simulink model "mpc_tgt_calc"  (R2025a)
settings: Solver=FixedStepDiscrete  StartTime=0.0  StopTime=2600  FixedStep=0.1  RelTol=1e-3
undefined symbols (not defined in the file): accl, alpha, alpha2, ang, beta, cnt_delay_accl_ratio, cnt_delay_decel_ratio, delay_accl, delay_v, dist, dt, ff_duty_front, ff_duty_l, ff_duty_r, ff_duty_roll, ff_duty_rpm_l, ff_duty_rpm_r, ff_friction_torque_l, ff_friction_torque_r, ff_front_torque, ff_roll_torque, ideal_point, img_ang, img_dist, kanayama_point, pivot_state, pos_x, pos_y, sla_param, slip, slip_point, state, trj_diff, v, vx, vy, w
libraries: simulink_extras x1
(part 1 of 3)
settings Model: Creator=nao12  LastModifiedBy=naoto
settings SolverCC: AlgebraicLoopSolver=TrustRegion
settings DataIOCC: SaveOutput=off  SignalLogging=off  DSMLogging=off  SaveTime=off  ReturnWorkspaceOutputs=off
settings OptimizationCC: StrengthReduction=on  PassReuseOutputArgsAs=Individual arguments  ZeroExternalMemoryAtStartup=off  ZeroInternalMemoryAtStartup=off  OptimizeBlockOrder=speed  OptimizationPriority=Speed  OptimizationCustomize=off  MultiThreadedLoops=on  AutoScheduleForLoops=on  EfficientTunableParamExpr=on
settings DebuggingCC: ParameterTunabilityLossMsg=error  UnconnectedInputMsg=warning  UnconnectedOutputMsg=warning  UnconnectedLineMsg=warning  ArithmeticOperatorsInVariantConditions=warning
settings ModelReferenceCC: EnableRefExpFcnMdlSchedulingChecks=on
settings SFSimCC: SimCustomHeaderCode="#include \"bus.h\""  SimUserIncludeDirs=../include/  MATLABDynamicMemAlloc=off  CustomCodeUndefinedFunction=UseInterfaceOnly  SimTargetLang=C++  SimDLTargetLibrary=mkl-dnn
settings RTWCC: SystemTargetFile=ert.tlc  GenCodeOnly=on  TemplateMakefile=ert_default_tmf  GenerateReport=on  RTWUseSimCustomCode=on  CustomHeaderCode="#include \"bus.h\""  CustomInclude=../include/  Toolchain=GNU gcc/g++ | gmake (64-bit Linux)  IncludeHyperlinkInReport=on  LaunchReport=on  TargetLang=C++  GenerateTraceInfo=on  GenerateTraceReport=on  GenerateTraceReportSl=on  GenerateTraceReportSf=on  GenerateTraceReportEml=on  GenerateCodeMetricsReport=on  GPUComputeCapability=3.5  DLArmComputeVersion=19.05  Description=Embedded Coder
settings CodeAppCC: GenerateComments=off  IgnoreCustomStorageClasses=off  OperatorAnnotations=on  SimulinkDataObjDesc=on  SFDataObjDesc=on  SimulinkBlockComments=off
settings ERTTargetCC: ExtModeTransport=0.0  ExtModeStaticAlloc=off  ExtModeMexFile=ext_comm  ExtModeIntrfLevel=Level1  InlinedParameterPlacement=Hierarchical  RootIOFormat=Structure reference  ERTCustomFileTemplate=example_file_process.tlc  DynamicArrayContainerType=coder::array  TargetLangStandard=C++11 (ISO)  GenerateSampleERTMain=on  SupportAbsoluteTime=off  CodeInterfacePackaging=C++ class  SupportComplex=off  ParenthesesLevel=Minimum
settings SimscapeCC: SimscapeLogDecimation=1  SimscapeLogDataHistory=5000

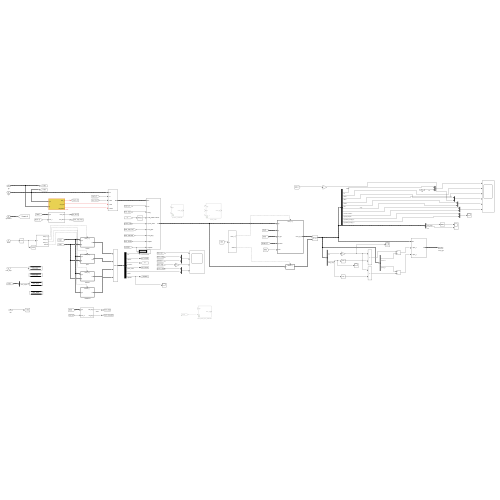
[thumbnail: Simulink's stored preview of the top-level diagram]
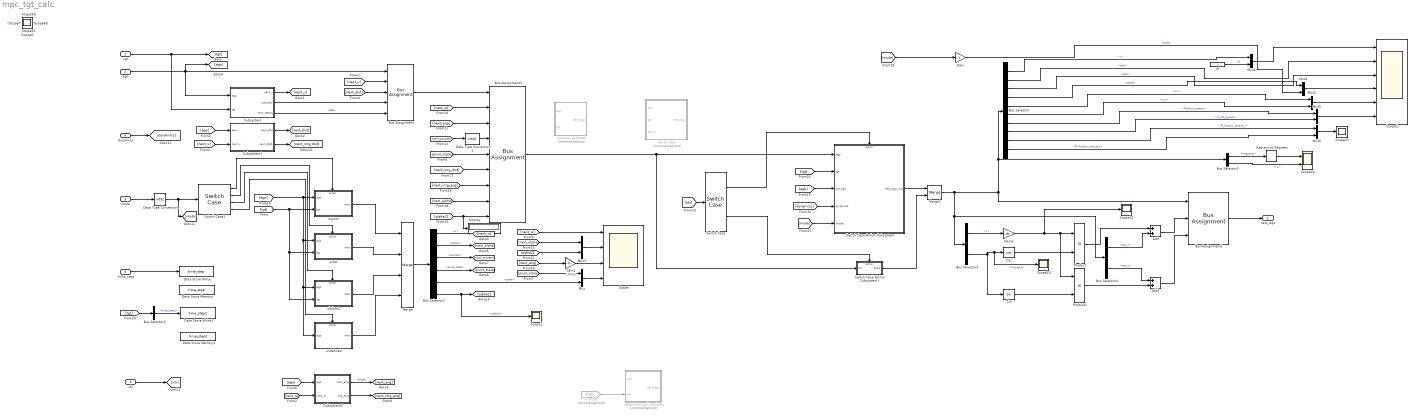
== system mpc_tgt_calc ==
  tgt : Inport  OutDataTypeStr=Bus: t_tgt  BusOutputAsStruct=on
  ego : Inport  Port=2  OutDataTypeStr=Bus: t_ego  BusOutputAsStruct=on
  mode : Inport  Port=3  OutDataTypeStr=int32
  time_step : Inport  Port=4  OutDataTypeStr=int32
  dynamics : Inport  Port=5  OutDataTypeStr=Bus: t_dynamics  BusOutputAsStruct=on
  idx : Inport  Port=6  OutDataTypeStr=int32
  Add : Sum
  Add1 : Sum
  Bus Assignment : BusAssignment  AssignedSignals=v,dist,accl,state
  Bus Assignment1 : BusAssignment  AssignedSignals=w,ang,sla_param.counter,pivot_state,img_dist,img_ang,alpha,alpha2
  Bus Assignment2 : BusAssignment  AssignedSignals=pos_x,pos_y
  Bus Selector : BusSelector  OutputSignals=v,accl,dist,state,slip.vx,slip.vy,ff_front_torque,ff_roll_torque,ff_friction_torque_l,ff_friction_torque_r
  Bus Selector1 : BusSelector  OutputSignals=w,alpha,sla_param.counter,pivot_state,sla_param.state,alpha2
  Bus Selector2 : BusSelector  OutputSignals=time_step2
  Bus Selector3 : BusSelector  OutputSignals=v,img_ang
  Bus Selector4 : BusSelector  OutputSignals=pos_x,pos_y
  Bus Selector5 : BusSelector  OutputSignals=img_ang,w
  Cos : Trigonometry  Operator=cos
  Data Store Memory : DataStoreMemory  DataStoreName=time_step  ReadBeforeWriteMsg=warning  WriteAfterWriteMsg=warning  WriteAfterReadMsg=warning  ShowAdditionalParam=off
  Data Store Memory1 : DataStoreMemory  DataStoreName=time_step2  ReadBeforeWriteMsg=warning  WriteAfterWriteMsg=warning  WriteAfterReadMsg=warning  ShowAdditionalParam=off
  Data Store Write : DataStoreWrite  DataStoreName=time_step  IndexOptions=Index vector (dialog)  Indices=1  OutputSizes=1
  Data Store Write1 : DataStoreWrite  DataStoreName=time_step2  IndexOptions=Index vector (dialog)  Indices=1  OutputSizes=1
  Data Type Conversion : DataTypeConversion  OutDataTypeStr=int32  SaturateOnIntegerOverflow=off  RndMeth=Floor
  Data Type Conversion1 : DataTypeConversion  OutDataTypeStr=int32  SaturateOnIntegerOverflow=off  RndMeth=Floor
  Display : Display
  From19 : From  Commented=on  GotoTag=tgt
  Gain : Gain  OutDataTypeStr=int32
  Gain1 : Gain  Gain=180/pi
  Gain2 : Gain  Gain=dt
  Merge : Merge  Inputs=4
  Merge1 : Merge
  Mux{,1..6} (7 alike) : Mux  Inputs=2
  Product : Product
  Product1 : Product
  Radians to Degrees : simulink_extras/Transformations/Radians to Degrees
  Scope : Scope  NumInputPorts=4
      settings: ActiveDisplayYMinimum=-2.63908  ActiveDisplayYMaximum=23.74994  DataLoggingVariableName=ScopeData2
  Scope{1,3..19,21..23} (21 alike) : Scope
      Scope1 settings: ActiveDisplayYMinimum=-2973.3984756469727  ActiveDisplayYMaximum=1247.0022964477539  DataLoggingVariableName=ScopeData2
      Scope21 settings: ActiveDisplayYMinimum=0.0163018349558115  ActiveDisplayYMaximum=0.017838163301348686
      Scope22 settings: ActiveDisplayYMinimum=0.20000004768371582  ActiveDisplayYMaximum=2.2000000476837158  DataLoggingVariableName=ScopeData10
      Scope23 settings: ActiveDisplayYMinimum=0.20000004768371582  ActiveDisplayYMaximum=2.2000000476837158  DataLoggingVariableName=ScopeData11
      Scope10 settings: ActiveDisplayYMinimum=0.5708  ActiveDisplayYMaximum=2.5708  DataLoggingVariableName=ScopeData3
      Scope11 settings: ActiveDisplayYMinimum=-360.06396  ActiveDisplayYMaximum=3240.57568  DataLoggingVariableName=ScopeData4
      Scope12 settings: ActiveDisplayYMinimum=1880  ActiveDisplayYMaximum=3880  DataLoggingVariableName=ScopeData5
      Scope13 settings: ActiveDisplayYMinimum=-0.97134  ActiveDisplayYMaximum=-0.37241  DataLoggingVariableName=ScopeData6
      Scope14 settings: ActiveDisplayYMinimum=-11.26948  ActiveDisplayYMaximum=1.25216  DataLoggingVariableName=ScopeData7
      Scope15 settings: DataLoggingVariableName=ScopeData8
      Scope16 settings: ActiveDisplayYMinimum=-1  ActiveDisplayYMaximum=1  DataLoggingVariableName=ScopeData9
      Scope17 settings: ActiveDisplayYMinimum=-22.53325  ActiveDisplayYMaximum=202.50369
      Scope18 settings: ActiveDisplayYMinimum=-1  ActiveDisplayYMaximum=1
      Scope19 settings: ActiveDisplayYMinimum=-0.125  ActiveDisplayYMaximum=1.125  DataLoggingVariableName=ScopeData2
      Scope3 settings: ActiveDisplayYMinimum=-11  ActiveDisplayYMaximum=-9  DataLoggingVariableName=ScopeData4
      Scope4 settings: ActiveDisplayYMinimum=-11  ActiveDisplayYMaximum=-9  DataLoggingVariableName=ScopeData5
      Scope5 settings: ActiveDisplayYMinimum=-11  ActiveDisplayYMaximum=-9  DataLoggingVariableName=ScopeData6
      Scope6 settings: ActiveDisplayYMinimum=9  ActiveDisplayYMaximum=11  DataLoggingVariableName=ScopeData7
      Scope7 settings: ActiveDisplayYMinimum=-1  ActiveDisplayYMaximum=1  DataLoggingVariableName=ScopeData8
      Scope8 settings: ActiveDisplayYMinimum=-0.25  ActiveDisplayYMaximum=2.25
      Scope9 settings: ActiveDisplayYMinimum=0.0004  ActiveDisplayYMaximum=0.0006  DataLoggingVariableName=ScopeData2
  Scope2 : Scope  NumInputPorts=6
      settings: ActiveDisplayYMinimum=-724.5  ActiveDisplayYMaximum=6520.5
  Scope20 : Scope  NumInputPorts=2
      settings: ActiveDisplayYMinimum=-5.62498  ActiveDisplayYMaximum=50.64557  DataLoggingVariableName=ScopeData2
  Sin : Trigonometry
  Subsystem : Subsystem
  Subsystem1 : Subsystem
  Subsystem3 : Subsystem
  Switch Case : SwitchCase
  Switch Case Action Subsystem : Subsystem  TreatAsAtomicUnit=on
  Switch Case Action Subsystem1 : Subsystem  TreatAsAtomicUnit=on
  Switch Case1 : SwitchCase  CaseConditions={1,2,4}
  decel_ratio : Subsystem  Commented=on
  kanayama_ctrl_method1 : Subsystem  Commented=on
  pivot : Subsystem  TreatAsAtomicUnit=on
  position_estimate : Subsystem  Commented=on
  slalom : Subsystem  TreatAsAtomicUnit=on
  slalom2 : Subsystem  TreatAsAtomicUnit=on
  undefined : Subsystem  TreatAsAtomicUnit=on
  v0 : Constant  Value=0  OutDataTypeStr=single
  next_ego : Outport  OutDataTypeStr=Bus: t_ego
  wires:
  mode/1 -> Data Type Conversion/1
  tgt/1 -> [tgt], Subsystem/2(tgt)
  ego/1 -> Subsystem/1(ego), Bus Assignment/1, [ego]
  Data Type Conversion/1 -> [mode], Switch Case1/1
  Switch Case1/1 -> slalom/Action
  [tgt] -> slalom2/2(tgt), pivot/2(tgt), slalom/2(tgt)
  Bus Assignment/1 -> Bus Assignment1/1
  [next_v] -> Bus Assignment/2
  [next_dist] -> Bus Assignment/3
  Subsystem/1(next_v) -> [next_v]
  [next_v] -> Subsystem1/2(next_v)
  Subsystem1/1(next_dist) -> [next_dist]
  Subsystem/2(use_accl) -> Bus Assignment/4
  Subsystem/3(next_status) -> Bus Assignment/5  "state"
  [next_w] -> Subsystem3/2(next_w)
  [ego] -> Subsystem1/1(ego)
  [ego] -> Subsystem3/1(ego)
  Subsystem3/1(next_ang) -> [next_ang]  "angle"
  Bus Selector/4 -> Mux4/1  "<state>"
  Bus Selector/3 -> Scope2/3  "<dist>"
  [next_w] -> Bus Assignment1/2
  [next_ang] -> Bus Assignment1/3
  [next_counter] -> Data Type Conversion1/1
  Data Type Conversion1/1 -> Bus Assignment1/4
  [next_w] -> Scope/1
  [next_ang] -> Gain1/1
  Switch Case1/2 -> pivot/Action
  [ego] -> slalom2/1(ego), undefined/1(ego), pivot/1(ego), slalom/1(ego)
  Switch Case1/4 -> undefined/Action
  Merge/1 -> Bus Selector1/1
  Bus Selector1/1 -> [next_w]  "<w>"
  Bus Selector1/2 -> [next_alpha]  "<alpha>"
  Bus Selector1/3 -> [next_counter]  "<counter>"
  slalom/1(next) -> Merge/1
  pivot/1(next) -> Merge/2
  undefined/1(next) -> Merge/4
  Bus Selector1/4 -> [pivot_state]  "<pivot_state>"
  [pivot_state] -> Bus Assignment1/5
  Mux/1 -> Scope/4
  [pivot_state] -> Mux/1
  Bus Selector1/5 -> Mux/2  "<state>"
  Subsystem3/2(img_ang) -> [next_img_ang]
  [next_img_ang] -> Bus Assignment1/7
  Subsystem1/2(next_dist1) -> [next_img_dist]
  [next_img_dist] -> Bus Assignment1/6
  [next_alpha] -> Bus Assignment1/8
  From19/1 -> kanayama_ctrl_method1/2(tgt)
  time_step/1 -> Data Store Write/1
  slalom2/1(next) -> Merge/3
  Switch Case1/3 -> slalom2/Action
  Mux1/1 -> Scope2/1
  Bus Selector/1 -> Mux1/1  "<v>"
  v0/1 -> Mux1/2  "v0"
  dynamics/1 -> [dynamics]
  Bus Selector2/1 -> Data Store Write1/1  "<time_step2>"
  [tgt] -> Bus Selector2/1
  Bus Selector1/6 -> Scope1/1, [alpha2]  "<alpha2>"
  Mux3/1 -> Scope/2
  [next_alpha] -> Mux3/1
  [alpha2] -> Mux3/2
  [alpha2] -> Display/1, Bus Assignment1/9
  [mode] -> Gain/1
  Gain/1 -> Mux4/2  "mode"
  Bus Selector/2 -> Scope2/2  "<accl>"
  Bus Selector/5 -> Mux2/1  "<vx>"
  Bus Selector/6 -> Mux2/2  "<vy>"
  Mux2/1 -> Scope2/5
  Gain1/1 -> Scope/3
  Bus Selector5/1 -> Radians to Degrees/1  "<img_ang>"
  Bus Selector5/2 -> Scope20/2  "<w>"
  Radians to Degrees/1 -> Scope20/1
  Mux4/1 -> Scope2/4
  Mux5/1 -> Scope2/6
  Bus Selector/7 -> Mux5/1  "<ff_front_torque>"
  Bus Selector/8 -> Mux5/2  "<ff_roll_torque>"
  Bus Selector/9 -> Mux6/1  "<ff_friction_torque_l>"
  Bus Selector/10 -> Mux6/2  "<ff_friction_torque_r>"
  Mux6/1 -> Scope21/1
  idx/1 -> [idx]
  Merge1/1 -> Bus Selector4/1, Bus Selector3/1, Bus Selector/1, Bus Selector5/1, Bus Assignment2/1
  Bus Assignment1/1 -> Switch Case Action Subsystem/1(ego), Switch Case Action Subsystem1/1(In1)
  [tgt] -> Switch Case Action Subsystem/2(tgt)
  [ego] -> Switch Case Action Subsystem/3(old_ego)
  [dynamics] -> Switch Case Action Subsystem/4(dynamics)
  [mode] -> Switch Case Action Subsystem/5(mode)
  [idx] -> Switch Case/1
  Switch Case/1 -> Switch Case Action Subsystem/Action
  Switch Case Action Subsystem1/1(Out1) -> Merge1/2
  Switch Case Action Subsystem/1(next_ego_out) -> Merge1/1
  Switch Case/2 -> Switch Case Action Subsystem1/Action
  Bus Selector3/1 -> Gain2/1  "<v>"
  Bus Selector3/2 -> Sin/1, Scope23/1, Cos/1  "<img_ang>"
  Cos/1 -> Product/2
  Gain2/1 -> Scope22/1, Product1/1, Product/1
  Sin/1 -> Product1/2
  Bus Selector4/1 -> Add/2  "<pos_x>"
  Bus Selector4/2 -> Add1/1  "<pos_y>"
  Product/1 -> Add/1
  Product1/1 -> Add1/2
  Bus Assignment2/1 -> next_ego/1
  Add/1 -> Bus Assignment2/2
  Add1/1 -> Bus Assignment2/3

== system mpc_tgt_calc/Subsystem ==
  ego : Inport
  tgt : Inport  Port=2
  Bus Selector2 : BusSelector  OutputSignals=v_max
  If : If  IfExpression=u1 >= 0
  Merge : Merge
  Merge1 : Merge
  Merge2 : Merge
  straight_ahead : Subsystem  TreatAsAtomicUnit=on
  straight_back : Subsystem  TreatAsAtomicUnit=on
  next_v : Outport
  use_accl : Outport  Port=2
  next_status : Outport  Port=3
  wires:
  tgt/1 -> [tgt], Bus Selector2/1
  Bus Selector2/1 -> If/1  "<v_max>"
  If/1 -> straight_ahead/Action
  ego/1 -> [ego]
  [ego] -> straight_ahead/1(ego)
  [tgt] -> straight_ahead/2(tgt)
  [ego] -> straight_back/1(ego)
  [tgt] -> straight_back/2(tgt)
  If/2 -> straight_back/Action
  straight_ahead/1(next_v) -> Merge/1
  straight_ahead/2(use_accl) -> Merge1/1
  straight_ahead/3(next_status) -> Merge2/1
  straight_back/1(next_v) -> Merge/2
  straight_back/2(use_accl) -> Merge1/2
  straight_back/3(next_status) -> Merge2/2
  Merge/1 -> next_v/1
  Merge1/1 -> use_accl/1
  Merge2/1 -> next_status/1

== system mpc_tgt_calc/Subsystem1 ==
  ego : Inport
  next_v : Inport  Port=2
  Add1 : Sum
  Add2 : Sum
  Bus Selector : BusSelector  OutputSignals=dist,img_dist
  Data Store Read : DataStoreRead  DataStoreName=time_step  IndexOptions=Index vector (dialog)  Indices=1  OutputSizes=1
  Data Type Conversion1 : DataTypeConversion  OutDataTypeStr=single  SaturateOnIntegerOverflow=off  RndMeth=Floor
  Data Type Conversion2 : DataTypeConversion  OutDataTypeStr=single  SaturateOnIntegerOverflow=off  RndMeth=Floor
  Data Type Conversion3 : DataTypeConversion  OutDataTypeStr=single  SaturateOnIntegerOverflow=off  RndMeth=Floor
  Gain1 : Gain  Gain=dt
  Product : Product
  next_dist : Outport
  next_dist1 : Outport  Port=2
  wires:
  ego/1 -> Bus Selector/1
  Bus Selector/1 -> Add1/1  "<dist>"
  Add1/1 -> Data Type Conversion1/1
  Data Type Conversion1/1 -> next_dist/1
  Add2/1 -> Data Type Conversion2/1
  Gain1/1 -> Add2/2, Add1/2
  Data Type Conversion2/1 -> next_dist1/1
  Bus Selector/2 -> Add2/1  "<img_dist>"
  Product/1 -> Gain1/1
  next_v/1 -> Product/1
  Data Store Read/1 -> Data Type Conversion3/1
  Data Type Conversion3/1 -> Product/2

== system mpc_tgt_calc/Subsystem3 ==
  ego : Inport
  next_w : Inport  Port=2
  Add1 : Sum
  Add2 : Sum
  Bus Selector : BusSelector  OutputSignals=ang,img_ang
  Data Store Read : DataStoreRead  DataStoreName=time_step  IndexOptions=Index vector (dialog)  Indices=1  OutputSizes=1
  Data Type Conversion1 : DataTypeConversion  OutDataTypeStr=single  SaturateOnIntegerOverflow=off  RndMeth=Floor
  Data Type Conversion2 : DataTypeConversion  OutDataTypeStr=single  SaturateOnIntegerOverflow=off  RndMeth=Floor
  Data Type Conversion3 : DataTypeConversion  OutDataTypeStr=single  SaturateOnIntegerOverflow=off  RndMeth=Floor
  Gain1 : Gain  Gain=dt
  Product : Product
  next_ang : Outport
  img_ang : Outport  Port=2
  wires:
  ego/1 -> Bus Selector/1
  Add1/1 -> Data Type Conversion1/1
  Bus Selector/1 -> Add1/1  "<ang>"
  Data Type Conversion1/1 -> next_ang/1
  Bus Selector/2 -> Add2/1  "<img_ang>"
  Data Type Conversion2/1 -> img_ang/1
  Add2/1 -> Data Type Conversion2/1
  Gain1/1 -> Add1/2, Add2/2
  Data Store Read/1 -> Data Type Conversion3/1
  Product/1 -> Gain1/1
  next_w/1 -> Product/1
  Data Type Conversion3/1 -> Product/2

== system mpc_tgt_calc/Switch Case Action Subsystem ==
  ego : Inport
  tgt : Inport  Port=2
  old_ego : Inport  Port=3
  dynamics : Inport  Port=4
  mode : Inport  Port=5
  Action Port : ActionPort  ActionPortLabel=case [ 1 ]:
  Bus Selector4 : BusSelector  OutputSignals=alpha2
  Bus Selector6 : BusSelector  OutputSignals=enable_slip_decel
  Constant4 : Constant  OutDataTypeStr=int8
  Display1 : Display
  If1 : If  IfExpression=u1 == 1
  Logical Operator3 : Logic  AllPortsSameDT=off  OutDataTypeStr=boolean
  Merge1 : Merge
  calc_FF : Subsystem
  no_slip : Subsystem  TreatAsAtomicUnit=on
  slip decel : Subsystem  TreatAsAtomicUnit=on
  next_ego_out : Outport
  wires:
  dynamics/1 -> [dynamics], slip decel/4(dynamics)
  [dynamics] -> calc_FF/2(dynamics)
  Bus Selector6/1 -> Logical Operator3/2  "<enable_slip_decel>"
  [mode] -> calc_FF/3(mode)
  calc_FF/1(next_ego_out) -> next_ego_out/1
  [ego] -> calc_FF/4(ego_z)
  old_ego/1 -> [ego], slip decel/3(old_ego)
  Logical Operator3/1 -> If1/1
  Constant4/1 -> Logical Operator3/1
  Merge1/1 -> Bus Selector4/1, calc_FF/1(next_ego)
  mode/1 -> [mode]
  slip decel/1(next) -> Merge1/1
  tgt/1 -> slip decel/2(tgt), Bus Selector6/1
  ego/1 -> no_slip/1(ego), slip decel/1(ego)
  If1/2 -> no_slip/Action
  no_slip/1(next) -> Merge1/2
  Bus Selector4/1 -> Display1/1  "<alpha2>"
  If1/1 -> slip decel/Action

== system mpc_tgt_calc/Switch Case Action Subsystem1 ==
  In1 : Inport
  Action Port : ActionPort  ActionPortLabel=default:
  Out1 : Outport
  wires:
  In1/1 -> Out1/1

== system mpc_tgt_calc/decel_ratio ==
  ego : Inport
  tgt : Inport  Port=2
  ego_z : Inport  Port=3
  Bus Assignment : BusAssignment  AssignedSignals=delay_v,delay_accl,cnt_delay_accl_ratio,cnt_delay_decel_ratio
  Bus Selector : BusSelector  OutputSignals=accl
  Bus Selector1 : BusSelector  OutputSignals=v
  Data Store Read : DataStoreRead  DataStoreName=time_step  IndexOptions=Index vector (dialog)  Indices=1  OutputSizes=1
  Gain : Gain  Gain=dt
  If : If  ElseIfExpressions=u1 < 0
  If Action Subsystem : Subsystem  TreatAsAtomicUnit=on
  If Action Subsystem1 : Subsystem  TreatAsAtomicUnit=on
  If Action Subsystem2 : Subsystem  TreatAsAtomicUnit=on
  Merge : Merge  Inputs=3
  Merge1 : Merge  Inputs=3
  Merge2 : Merge  Inputs=3
  Product : Product
  next_ego : Outport
  wires:
  Bus Assignment/1 -> next_ego/1
  If/1 -> If Action Subsystem/Action
  ego/1 -> [ego], Bus Selector/1, Bus Assignment/1
  [ego] -> If Action Subsystem/1(ego)
  Bus Selector/1 -> If/1  "<accl>"
  tgt/1 -> If Action Subsystem/2(tgt), If Action Subsystem1/2(tgt)
  If/2 -> If Action Subsystem1/Action
  If/3 -> If Action Subsystem2/Action
  [ego] -> If Action Subsystem1/1(ego)
  If Action Subsystem/1(ff_accl) -> Merge/1
  If Action Subsystem1/1(ff_accl) -> Merge/2
  If Action Subsystem2/1(ff_accl) -> Merge/3
  If Action Subsystem/2(cnt_delay_accl_ratio) -> Merge1/1
  If Action Subsystem1/2(cnt_delay_accl_ratio) -> Merge1/2
  If Action Subsystem2/2(cnt_delay_accl_ratio) -> Merge1/3
  If Action Subsystem/3(cnt_delay_decel_ratio) -> Merge2/1
  If Action Subsystem1/3(cnt_delay_decel_ratio) -> Merge2/2
  If Action Subsystem2/3(cnt_delay_decel_ratio) -> Merge2/3
  Merge/1 -> Bus Assignment/3
  Merge1/1 -> Bus Assignment/4
  Merge2/1 -> Bus Assignment/5
  [ego] -> If Action Subsystem2/1(ego)
  ego_z/1 -> Bus Selector1/1
  Data Store Read/1 -> Product/1
  Gain/1 -> Product/2
  Bus Selector1/1 -> Gain/1  "<v>"
  Product/1 -> Bus Assignment/2

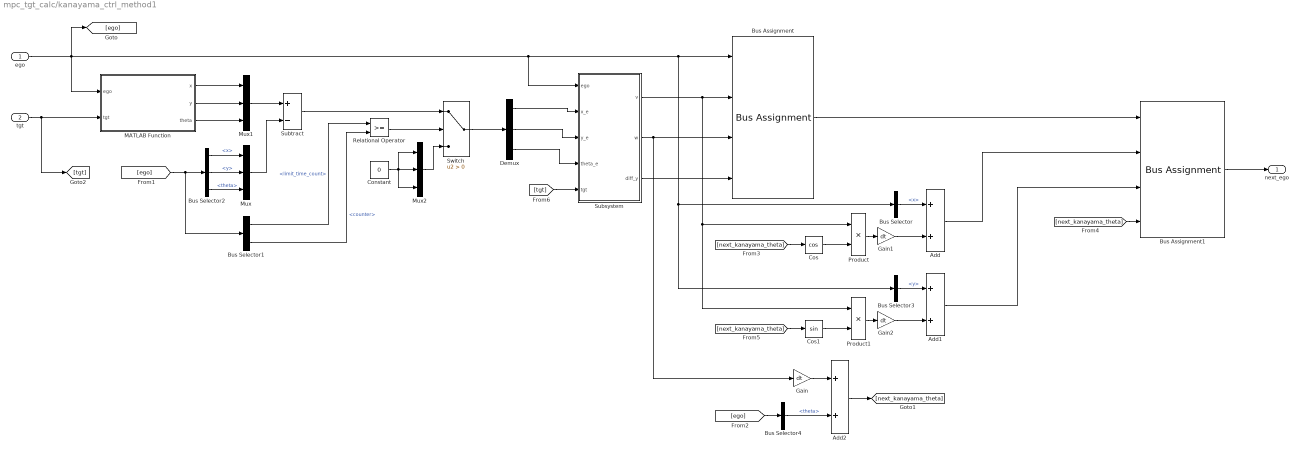
== system mpc_tgt_calc/kanayama_ctrl_method1 ==
  ego : Inport
  tgt : Inport  Port=2
  Add : Sum
  Add1 : Sum
  Add2 : Sum
  Bus Assignment : BusAssignment  AssignedSignals=kanayama_point.v,kanayama_point.w,kanayama_point.y
  Bus Assignment1 : BusAssignment  AssignedSignals=kanayama_point.x,kanayama_point.y,kanayama_point.theta
  Bus Selector : BusSelector  OutputSignals=kanayama_point.x
  Bus Selector1 : BusSelector  OutputSignals=sla_param.limit_time_count,sla_param.counter
  Bus Selector2 : BusSelector  OutputSignals=slip_point.x,slip_point.y,slip_point.theta
  Bus Selector3 : BusSelector  OutputSignals=kanayama_point.y
  Bus Selector4 : BusSelector  OutputSignals=kanayama_point.theta
  Constant : Constant  Value=0  OutDataTypeStr=single
  Cos : Trigonometry  Operator=cos
  Cos1 : Trigonometry
  Demux : Demux  Outputs=3
  Gain : Gain  Gain=dt
  Gain1 : Gain  Gain=dt
  Gain2 : Gain  Gain=dt
  MATLAB Function : MATLAB Function  TreatAsAtomicUnit=on
  Mux : Mux  Inputs=3
  Mux1 : Mux  Inputs=3
  Mux2 : Mux  Inputs=3
  Product : Product
  Product1 : Product
  Relational Operator : RelationalOperator  OutDataTypeStr=boolean  RndMeth=Simplest  InputSameDT=off
  Subsystem : Subsystem
  Subtract : Sum  Inputs=+-
  Switch : Switch  Criteria=u2 > Threshold  SaturateOnIntegerOverflow=off  InputSameDT=off
  next_ego : Outport
  wires:
  tgt/1 -> [tgt], MATLAB Function/2(tgt)
  Bus Selector2/1 -> Mux/1  "<x>"
  Bus Selector2/2 -> Mux/2  "<y>"
  Bus Selector2/3 -> Mux/3  "<theta>"
  MATLAB Function/1(x) -> Mux1/1
  MATLAB Function/2(y) -> Mux1/2
  MATLAB Function/3(theta) -> Mux1/3
  Mux1/1 -> Subtract/1
  Mux/1 -> Subtract/2
  Switch/1 -> Demux/1
  Bus Selector1/1 -> Relational Operator/1  "<limit_time_count>"
  Bus Selector1/2 -> Relational Operator/2  "<counter>"
  Relational Operator/1 -> Switch/2
  Subtract/1 -> Switch/1
  Mux2/1 -> Switch/3
  Constant/1 -> Mux2/1, Mux2/2, Mux2/3
  Bus Assignment/1 -> Bus Assignment1/1
  Demux/1 -> Subsystem/2(x_e)
  Demux/2 -> Subsystem/3(y_e)
  Demux/3 -> Subsystem/4(theta_e)
  Subsystem/2(w) -> Gain/1, Bus Assignment/3
  Product/1 -> Gain1/1
  Bus Selector/1 -> Add/1  "<x>"
  Add/1 -> Bus Assignment1/2
  Add1/1 -> Bus Assignment1/3
  Cos/1 -> Product/2
  Subsystem/1(v) -> Product/1, Product1/1, Bus Assignment/2
  [next_kanayama_theta] -> Cos/1
  Gain1/1 -> Add/2
  Cos1/1 -> Product1/2
  Gain2/1 -> Add1/2
  ego/1 -> MATLAB Function/1(ego), [ego], Subsystem/1(ego), Bus Selector3/1, Bus Selector/1, Bus Assignment/1
  Product1/1 -> Gain2/1
  Bus Assignment1/1 -> next_ego/1
  [ego] -> Bus Selector1/1, Bus Selector2/1
  [ego] -> Bus Selector4/1
  Gain/1 -> Add2/1
  Bus Selector4/1 -> Add2/2  "<theta>"
  Add2/1 -> [next_kanayama_theta]
  Bus Selector3/1 -> Add1/1  "<y>"
  [next_kanayama_theta] -> Bus Assignment1/4
  [next_kanayama_theta] -> Cos1/1
  [tgt] -> Subsystem/5(tgt)
  Subsystem/3(diff_y) -> Bus Assignment/4

== system mpc_tgt_calc/pivot ==
  ego : Inport
  tgt : Inport  Port=2
  Action Port : ActionPort  ActionPortLabel=case [ 2 ]:
  Abs : Abs  SaturateOnIntegerOverflow=off
  Abs1 : Abs  SaturateOnIntegerOverflow=off
  Add : Sum
  Bus Assignment : BusAssignment  AssignedSignals=w,alpha,alpha2,pivot_state
  Bus Assignment1 : BusAssignment  AssignedSignals=w,alpha,alpha2,pivot_state
  Bus Selector : BusSelector  OutputSignals=w
  Bus Selector1 : BusSelector  OutputSignals=ang
  Bus Selector2 : BusSelector  OutputSignals=tgt_angle
  Constant : Constant  Value=0  OutDataTypeStr=single
  Constant1 : Constant  Value=3  OutDataTypeStr=int32
  Data Store Read : DataStoreRead  DataStoreName=time_step  IndexOptions=Index vector (dialog)  Indices=1  OutputSizes=1
  Data Type Conversion1 : DataTypeConversion  OutDataTypeStr=single  SaturateOnIntegerOverflow=off  RndMeth=Floor
  Data Type Conversion2 : DataTypeConversion  OutDataTypeStr=single  SaturateOnIntegerOverflow=off  RndMeth=Floor
  Data Type Conversion3 : DataTypeConversion  OutDataTypeStr=single  SaturateOnIntegerOverflow=off  RndMeth=Floor
  Gain : Gain  Gain=dt
  Product : Product
  Relational Operator1 : RelationalOperator  Operator=<  OutDataTypeStr=boolean  RndMeth=Simplest  InputSameDT=off
  Subsystem : Subsystem
  Switch2 : Switch  Criteria=u2 > Threshold  SaturateOnIntegerOverflow=off  InputSameDT=off
  next : Outport
  wires:
  ego/1 -> Subsystem/1(ego), Bus Selector/1, Bus Assignment/1, [ego]
  Subsystem/1(next_alpha) -> Data Type Conversion1/1, Gain/1
  Bus Selector/1 -> Add/1  "<w>"
  Add/1 -> Data Type Conversion2/1
  Data Type Conversion2/1 -> Bus Assignment/2
  tgt/1 -> [tgt], Subsystem/2(tgt)
  Data Type Conversion1/1 -> Bus Assignment/4, Bus Assignment/3
  Subsystem/2(state_out) -> Bus Assignment/5
  Bus Assignment/1 -> Bus Assignment1/1, Switch2/1
  Relational Operator1/1 -> Switch2/2
  Bus Selector2/1 -> Abs1/1  "<tgt_angle>"
  Abs/1 -> Relational Operator1/1
  [ego] -> Bus Selector1/1
  [tgt] -> Bus Selector2/1
  Bus Selector1/1 -> Abs/1  "<ang>"
  Abs1/1 -> Relational Operator1/2
  Switch2/1 -> next/1
  Constant/1 -> Bus Assignment1/4, Bus Assignment1/3, Bus Assignment1/2
  Constant1/1 -> Bus Assignment1/5
  Bus Assignment1/1 -> Switch2/3
  Data Store Read/1 -> Data Type Conversion3/1
  Gain/1 -> Product/1
  Product/1 -> Add/2
  Data Type Conversion3/1 -> Product/2

== system mpc_tgt_calc/position_estimate ==
  ego : Inport
  tgt : Inport  Port=2
  Add : Sum
  Add1 : Sum
  Bus Assignment : BusAssignment  AssignedSignals=ideal_point.x,ideal_point.y,ideal_point.theta
  Bus Assignment1 : BusAssignment  AssignedSignals=trj_diff.x,trj_diff.y,trj_diff.theta
  Bus Selector : BusSelector  OutputSignals=ideal_point.x,v,img_ang
  Bus Selector1 : BusSelector  OutputSignals=ideal_point.y,v,img_ang
  Bus Selector2 : BusSelector  OutputSignals=ideal_point.theta
  Bus Selector3 : BusSelector  OutputSignals=ideal_point.x,ideal_point.y
  Bus Selector4 : BusSelector  OutputSignals=slip_point.x,slip_point.y
  Bus Selector5 : BusSelector  OutputSignals=img_ang,slip_point.theta
  Cos : Trigonometry  Operator=cos
  Cos1 : Trigonometry
  Data Store Read1 : DataStoreRead  DataStoreName=time_step  IndexOptions=Index vector (dialog)  Indices=1  OutputSizes=1
  Gain1 : Gain  Gain=dt
  Gain2 : Gain  Gain=dt
  Gain5 : Gain
  Gain6 : Gain
  Mux : Mux  Inputs=2
  Mux1 : Mux  Inputs=2
  Product{,1..3} (4 alike) : Product
  Scope : Scope  NumInputPorts=2
      settings: ActiveDisplayYMinimum=-25.25593  ActiveDisplayYMaximum=23.38566  DataLoggingVariableName=ScopeData2
  Subtract : Sum  Inputs=+-
  Subtract1 : Sum  Inputs=+-
  Subtract2 : Sum  Inputs=+-
  slipped_position_estimate : Subsystem
  next_ego : Outport
  wires:
  ego/1 -> slipped_position_estimate/1(ego), Bus Selector1/1, Bus Selector2/1, Bus Selector/1
  Bus Selector/1 -> Add/1  "<x>"
  Bus Selector/2 -> Product/1  "<v>"
  Bus Selector/3 -> Cos/1  "<img_ang>"
  Cos/1 -> Product/2
  Product/1 -> Gain1/1
  Bus Selector1/2 -> Product1/1  "<v>"
  Bus Selector1/1 -> Add1/1  "<y>"
  Product1/1 -> Gain2/1
  Bus Selector1/3 -> Cos1/1  "<img_ang>"
  Cos1/1 -> Product1/2
  Bus Selector2/1 -> Bus Assignment/4  "<theta>"
  Add1/1 -> Bus Assignment/3
  Add/1 -> Bus Assignment/2
  Bus Selector3/1 -> Subtract/1  "<x>"
  Bus Selector3/2 -> Subtract1/1  "<y>"
  slipped_position_estimate/1(next_ego) -> Bus Assignment/1
  Bus Selector4/1 -> Subtract/2  "<x>"
  Bus Selector4/2 -> Subtract1/2  "<y>"
  Subtract/1 -> Bus Assignment1/2, Mux1/1  "slip_diff_x"
  Subtract1/1 -> Mux1/2, Bus Assignment1/3  "slip_diff_y"
  Bus Assignment/1 -> Bus Selector5/1, Bus Selector3/1, Bus Assignment1/1, Bus Selector4/1
  Bus Selector5/2 -> Gain6/1  "<theta>"
  Gain6/1 -> Mux/2, Subtract2/2  "slipped_angle"
  Gain5/1 -> Mux/1, Subtract2/1  "ideal_angle"
  Bus Selector5/1 -> Gain5/1  "<img_ang>"
  Mux/1 -> Scope/2
  Mux1/1 -> Scope/1
  Bus Assignment1/1 -> next_ego/1
  Subtract2/1 -> Bus Assignment1/4  "slip_diff_theta"
  tgt/1 -> slipped_position_estimate/2(tgt)
  Product2/1 -> Add/2
  Gain1/1 -> Product2/1
  Product3/1 -> Add1/2
  Data Store Read1/1 -> Product3/1, Product2/2
  Gain2/1 -> Product3/2

== system mpc_tgt_calc/slalom ==
  ego : Inport
  tgt : Inport  Port=2
  Action Port : ActionPort  ActionPortLabel=case [ 1 ]:
  Bus Assignment : BusAssignment  AssignedSignals=w,alpha,sla_param.counter,alpha2
  Data Type Conversion : DataTypeConversion  OutDataTypeStr=int32  SaturateOnIntegerOverflow=off  RndMeth=Floor
  Data Type Conversion1 : DataTypeConversion  OutDataTypeStr=single  SaturateOnIntegerOverflow=off  RndMeth=Floor
  Data Type Conversion2 : DataTypeConversion  OutDataTypeStr=single  SaturateOnIntegerOverflow=off  RndMeth=Floor
  Data Type Conversion3 : DataTypeConversion  OutDataTypeStr=single  SaturateOnIntegerOverflow=off  RndMeth=Floor
  Subsystem2 : Subsystem
  next : Outport
  wires:
  ego/1 -> Subsystem2/1(ego), Bus Assignment/1
  tgt/1 -> Subsystem2/2(tgt)
  Bus Assignment/1 -> next/1
  Subsystem2/1(next_w) -> Data Type Conversion1/1
  Subsystem2/2(next_alpha) -> Data Type Conversion2/1
  Subsystem2/3(next_count) -> Data Type Conversion/1
  Data Type Conversion/1 -> Bus Assignment/4
  Data Type Conversion1/1 -> Bus Assignment/2
  Data Type Conversion2/1 -> Bus Assignment/3
  Data Type Conversion3/1 -> Bus Assignment/5
  Subsystem2/4(next_alpha2) -> Data Type Conversion3/1

== system mpc_tgt_calc/slalom2 ==
  ego : Inport
  tgt : Inport  Port=2
  Action Port : ActionPort  ActionPortLabel=case [ 4 ]:
  Abs : Abs  SaturateOnIntegerOverflow=off
  Abs1 : Abs  SaturateOnIntegerOverflow=off
  Add : Sum
  Bus Assignment : BusAssignment  AssignedSignals=w,alpha,pivot_state
  Bus Assignment1 : BusAssignment  AssignedSignals=w,alpha,alpha2,pivot_state
  Bus Selector : BusSelector  OutputSignals=w
  Bus Selector1 : BusSelector  OutputSignals=img_ang
  Bus Selector2 : BusSelector  OutputSignals=tgt_angle
  Bus Selector3 : BusSelector  OutputSignals=w
  Constant : Constant  Value=0  OutDataTypeStr=single
  Constant1 : Constant  Value=3  OutDataTypeStr=int32
  Data Store Read : DataStoreRead  DataStoreName=time_step  IndexOptions=Index vector (dialog)  Indices=1  OutputSizes=1
  Data Store Read1 : DataStoreRead  DataStoreName=time_step  IndexOptions=Index vector (dialog)  Indices=1  OutputSizes=1
  Data Type Conversion{1..4} (4 alike) : DataTypeConversion  OutDataTypeStr=single  SaturateOnIntegerOverflow=off  RndMeth=Floor
  Divide : Product  Inputs=*/
  Gain : Gain  Gain=dt
  Gain1 : Gain  Gain=dt
  Product : Product
  Relational Operator1 : RelationalOperator  Operator=<  OutDataTypeStr=boolean  RndMeth=Simplest  InputSameDT=off
  Scope : Scope
      settings: ActiveDisplayYMinimum=-1  ActiveDisplayYMaximum=1
  Subsystem : Subsystem
  Subtract : Sum  Inputs=+-
  Switch2 : Switch  Criteria=u2 > Threshold  SaturateOnIntegerOverflow=off  InputSameDT=off
  next : Outport
  wires:
  Subsystem/1(next_alpha) -> Data Type Conversion1/1, Gain/1
  Bus Selector/1 -> Add/1  "<w>"
  Add/1 -> Data Type Conversion2/1
  Data Type Conversion2/1 -> Bus Assignment/2
  Data Type Conversion1/1 -> Bus Assignment/3
  Subsystem/2(state_out) -> Bus Assignment/4
  Bus Assignment/1 -> Bus Assignment1/1, Switch2/1
  Relational Operator1/1 -> Switch2/2
  Bus Selector2/1 -> Abs1/1  "<tgt_angle>"
  Abs/1 -> Relational Operator1/1
  ego/1 -> Bus Selector3/1, Subsystem/1(ego), Bus Selector/1, Bus Selector1/1, Bus Assignment/1
  tgt/1 -> Bus Selector2/1, Subsystem/2(tgt)
  Bus Selector1/1 -> Abs/1  "<img_ang>"
  Abs1/1 -> Relational Operator1/2
  Switch2/1 -> next/1
  Constant1/1 -> Bus Assignment1/5
  Bus Assignment1/1 -> Switch2/3
  Data Store Read/1 -> Data Type Conversion3/1
  Gain/1 -> Product/1
  Product/1 -> Add/2
  Constant/1 -> Subtract/1, Bus Assignment1/4, Bus Assignment1/3, Bus Assignment1/2
  Bus Selector3/1 -> Subtract/2  "<w>"
  Subtract/1 -> Divide/1
  Data Store Read1/1 -> Data Type Conversion4/1
  Gain1/1 -> Divide/2
  Data Type Conversion3/1 -> Product/2
  Data Type Conversion4/1 -> Gain1/1

== system mpc_tgt_calc/undefined ==
  ego : Inport
  Action Port : ActionPort  ActionPortLabel=default:
  Bus Assignment1 : BusAssignment  AssignedSignals=w,alpha,alpha2
  Bus Selector3 : BusSelector  OutputSignals=w
  Constant : Constant  Value=0  OutDataTypeStr=single
  Data Store Read : DataStoreRead  DataStoreName=time_step  IndexOptions=Index vector (dialog)  Indices=1  OutputSizes=1
  Data Type Conversion1 : DataTypeConversion  OutDataTypeStr=single  SaturateOnIntegerOverflow=off  RndMeth=Floor
  Data Type Conversion2 : DataTypeConversion  OutDataTypeStr=single  SaturateOnIntegerOverflow=off  RndMeth=Floor
  Divide : Product  Inputs=*/
  Gain : Gain  Gain=dt
  Subtract : Sum  Inputs=+-
  next : Outport
  wires:
  ego/1 -> Bus Selector3/1, Bus Assignment1/1
  Gain/1 -> Divide/2
  Bus Selector3/1 -> Subtract/2  "<w>"
  Subtract/1 -> Divide/1
  Constant/1 -> Subtract/1, Bus Assignment1/2
  Divide/1 -> Bus Assignment1/4, Bus Assignment1/3
  Bus Assignment1/1 -> next/1
  Data Store Read/1 -> Data Type Conversion1/1
  Data Type Conversion1/1 -> Gain/1

== system mpc_tgt_calc/Subsystem/straight_ahead ==
  ego : Inport
  tgt : Inport  Port=2
  Action Port : ActionPort  ActionPortLabel=if(u1 >= 0)
  Add : Sum
  Bus Selector : BusSelector  OutputSignals=v
  Bus Selector1 : BusSelector  OutputSignals=v_max
  Constant : Constant  Value=0  OutDataTypeStr=single
  Data Store Read : DataStoreRead  DataStoreName=time_step  IndexOptions=Index vector (dialog)  Indices=1  OutputSizes=1
  Data Type Conversion1 : DataTypeConversion  OutDataTypeStr=single  SaturateOnIntegerOverflow=off  RndMeth=Floor
  Data Type Conversion2 : DataTypeConversion  OutDataTypeStr=single  SaturateOnIntegerOverflow=off  RndMeth=Floor
  Gain : Gain  Gain=dt
  Max : MinMax  Function=max  Inputs=2
  Min : MinMax  Inputs=2
  Product : Product
  Subsystem : Subsystem
  Unit Delay : UnitDelay  SampleTime=-1  HasFrameUpgradeWarning=on
  next_v : Outport
  use_accl : Outport  Port=2
  next_status : Outport  Port=3
  wires:
  Max/1 -> next_v/1
  Subsystem/1(use_accl) -> use_accl/1, Gain/1
  Constant/1 -> Max/2
  Bus Selector/1 -> Add/1  "<v>"
  ego/1 -> Subsystem/1(ego), Bus Selector/1
  tgt/1 -> Subsystem/2(tgt), Bus Selector1/1
  Data Type Conversion2/1 -> Min/2
  Min/1 -> Max/1  "velocity"
  Bus Selector1/1 -> Min/1  "<v_max>"
  Subsystem/2(next_state) -> next_status/1
  Add/1 -> Data Type Conversion2/1
  Data Store Read/1 -> Data Type Conversion1/1
  Product/1 -> Add/2
  Gain/1 -> Product/2
  Data Type Conversion1/1 -> Product/1
  Subsystem/3(cnt_out) -> Unit Delay/1
  Unit Delay/1 -> Subsystem/3(cnt_in)

== system mpc_tgt_calc/Subsystem/straight_back ==
  ego : Inport
  tgt : Inport  Port=2
  Action Port : ActionPort  ActionPortLabel=else
  Add : Sum
  Bus Selector : BusSelector  OutputSignals=v
  Bus Selector1 : BusSelector  OutputSignals=v_max
  Constant : Constant  Value=0  OutDataTypeStr=single
  Data Store Read : DataStoreRead  DataStoreName=time_step  IndexOptions=Index vector (dialog)  Indices=1  OutputSizes=1
  Data Type Conversion1 : DataTypeConversion  OutDataTypeStr=single  SaturateOnIntegerOverflow=off  RndMeth=Floor
  Data Type Conversion2 : DataTypeConversion  OutDataTypeStr=single  SaturateOnIntegerOverflow=off  RndMeth=Floor
  Gain : Gain  Gain=dt
  Max : MinMax  Inputs=2
  Min : MinMax  Function=max  Inputs=2
  Product : Product
  Subsystem : Subsystem
  next_v : Outport
  use_accl : Outport  Port=2
  next_status : Outport  Port=3
  wires:
  Max/1 -> next_v/1
  Subsystem/1(use_accl) -> use_accl/1, Gain/1
  Constant/1 -> Max/2
  Bus Selector/1 -> Add/1  "<v>"
  ego/1 -> Subsystem/1(ego), Bus Selector/1
  tgt/1 -> Subsystem/2(tgt), Bus Selector1/1
  Data Type Conversion2/1 -> Min/2
  Min/1 -> Max/1  "velocity"
  Bus Selector1/1 -> Min/1  "<v_max>"
  Subsystem/2(next_state) -> next_status/1
  Add/1 -> Data Type Conversion2/1
  Data Store Read/1 -> Data Type Conversion1/1
  Product/1 -> Add/2
  Gain/1 -> Product/2
  Data Type Conversion1/1 -> Product/1

== system mpc_tgt_calc/Switch Case Action Subsystem/calc_FF ==
  next_ego : Inport
  dynamics : Inport  Port=2
  mode : Inport  Port=3
  ego_z : Inport  Port=4
  Add : Sum  Inputs=+-+
  Add1 : Sum  Inputs=+++
  Bus Assignment : BusAssignment  AssignedSignals=ff_duty_front,ff_duty_l,ff_duty_r,ff_duty_roll,ff_duty_rpm_r,ff_duty_rpm_l,ff_front_torque,ff_roll_torque,ff_friction_torque_l,ff_friction_torque_r
  Mux : Mux  Inputs=2
  Mux1 : Mux  Inputs=2
  Scope : Scope  NumInputPorts=4
      settings: ActiveDisplayYMinimum=-56.35879  ActiveDisplayYMaximum=59.48451
  Scope1 : Scope
      settings: ActiveDisplayYMinimum=-54.68219  ActiveDisplayYMaximum=22.93296
  Subsystem : Subsystem
  calc_FF_Front : Subsystem
  calc_FF_Roll : Subsystem
  calc_counter_volt : Subsystem
  calc_counter_volt1 : Subsystem
  validation : Subsystem
  next_ego_out : Outport
  wires:
  next_ego/1 -> validation/1(next_ego)
  Bus Assignment/1 -> next_ego_out/1
  dynamics/1 -> calc_FF_Front/2(dynamics), calc_FF_Roll/2(dynamics), calc_counter_volt1/2(dynamics), calc_counter_volt/2(dynamics)
  calc_counter_volt/1(left) -> [rpm_l_volt], Mux/1, Add/3  "rpm_l_volt"
  calc_counter_volt/2(right) -> Add1/3, [rpm_r_volt], Mux/2  "rpm_r_volt"
  Mux/1 -> Scope/4
  calc_FF_Front/1(front_volt) -> Subsystem/2(front_volt)
  calc_FF_Roll/1(roll_volt) -> Scope1/1, Add1/2, Add/2, Scope/3, [roll_volt]
  Add1/1 -> Mux1/2, Bus Assignment/4  "FF_Right"
  Mux1/1 -> Scope/1
  Add/1 -> Mux1/1, Bus Assignment/3  "FF_Left"
  mode/1 -> Subsystem/3(mode)
  Subsystem/1(ff_front) -> Scope/2, Add1/1, Add/1, Bus Assignment/2
  validation/1(next_ego_out) -> calc_FF_Front/1(next_ego), calc_FF_Roll/1(next_ego), calc_counter_volt1/1(next_ego), calc_counter_volt/1(next_ego), Subsystem/1(next_ego), Bus Assignment/1
  ego_z/1 -> validation/2(ego_z)
  [roll_volt] -> Bus Assignment/5
  [rpm_r_volt] -> Bus Assignment/6
  [rpm_l_volt] -> Bus Assignment/7
  calc_FF_Front/2(front_torq) -> [front_torq]
  calc_FF_Roll/2(roll_torq) -> [roll_torq]
  [front_torq] -> Bus Assignment/8
  [roll_torq] -> Bus Assignment/9
  calc_counter_volt1/1(left) -> [friction_torque_l]  "rpm_l_volt"
  calc_counter_volt1/2(right) -> [friction_torque_r]  "rpm_r_volt"
  [friction_torque_l] -> Bus Assignment/10
  [friction_torque_r] -> Bus Assignment/11

== system mpc_tgt_calc/Switch Case Action Subsystem/no_slip ==
  ego : Inport
  Action Port : ActionPort  ActionPortLabel=else
  Bus Assignment : BusAssignment  AssignedSignals=beta,vx,vy,v
  Bus Assignment1 : BusAssignment  AssignedSignals=slip
  Bus Selector : BusSelector  OutputSignals=slip,v
  Constant : Constant  Value=0  OutDataTypeStr=single
  Gain : Gain  Gain=0.001
  Gain1 : Gain  Gain=0.001
  next : Outport
  wires:
  Bus Assignment1/1 -> next/1
  Bus Selector/1 -> Bus Assignment/1  "<slip>"
  ego/1 -> Bus Selector/1, Bus Assignment1/1
  Bus Assignment/1 -> Bus Assignment1/2
  Constant/1 -> Bus Assignment/4, Bus Assignment/2
  Bus Selector/2 -> Gain/1, Gain1/1  "<v>"
  Gain/1 -> Bus Assignment/5
  Gain1/1 -> Bus Assignment/3

== system mpc_tgt_calc/Switch Case Action Subsystem/slip decel ==
  ego : Inport
  tgt : Inport  Port=2
  old_ego : Inport  Port=3
  dynamics : Inport  Port=4
  Action Port : ActionPort  ActionPortLabel=if(u1 == 1)
  Bus Assignment1 : BusAssignment  AssignedSignals=slip,v,accl
  Bus Selector3 : BusSelector  OutputSignals=v
  Subsystem : Subsystem
  next : Outport
  wires:
  ego/1 -> Subsystem/1(next_ego), Bus Assignment1/1
  Bus Assignment1/1 -> next/1
  old_ego/1 -> Bus Selector3/1
  Subsystem/1(slip_param) -> Bus Assignment1/2
  tgt/1 -> Subsystem/2(tgt)
  Bus Selector3/1 -> Subsystem/3(old_v)  "<v>"
  Subsystem/2(v) -> Bus Assignment1/3
  Subsystem/3(accl) -> Bus Assignment1/4
  dynamics/1 -> Subsystem/4(dynamics)

== system mpc_tgt_calc/decel_ratio/If Action Subsystem ==
  ego : Inport
  tgt : Inport  Port=2
  Action Port : ActionPort  ActionPortLabel=if(u1 > 0)
  Add : Sum
  Bus Selector : BusSelector  OutputSignals=cnt_delay_accl_ratio,cnt_delay_decel_ratio
  Bus Selector1 : BusSelector  OutputSignals=accl
  Bus Selector2 : BusSelector  OutputSignals=limit_accl_ratio_cnt
  Constant : Constant  OutDataTypeStr=single
  Constant1 : Constant  OutDataTypeStr=single
  Divide : Product  Inputs=*/
  Product : Product
  Saturation : Saturate  UpperLimit=1  LowerLimit=0
  Switch : Switch  Criteria=u2 ~= 0  SaturateOnIntegerOverflow=off  InputSameDT=off
  ff_accl : Outport
  cnt_delay_accl_ratio : Outport  Port=2
  cnt_delay_decel_ratio : Outport  Port=3
  wires:
  ego/1 -> Bus Selector1/1, Bus Selector/1
  Bus Selector/1 -> Add/1  "<cnt_delay_accl_ratio>"
  Constant/1 -> Add/2
  Bus Selector/2 -> cnt_delay_decel_ratio/1  "<cnt_delay_decel_ratio>"
  Add/1 -> cnt_delay_accl_ratio/1, Divide/1
  tgt/1 -> Bus Selector2/1
  Divide/1 -> Saturation/1
  Saturation/1 -> Product/2
  Product/1 -> ff_accl/1
  Bus Selector1/1 -> Product/1  "<accl>"
  Constant1/1 -> Switch/3
  Bus Selector2/1 -> Switch/2, Switch/1  "<limit_accl_ratio_cnt>"
  Switch/1 -> Divide/2

== system mpc_tgt_calc/decel_ratio/If Action Subsystem1 ==
  ego : Inport
  tgt : Inport  Port=2
  Action Port : ActionPort  ActionPortLabel=elseif(u1 < 0)
  Add : Sum
  Bus Selector : BusSelector  OutputSignals=cnt_delay_decel_ratio,cnt_delay_accl_ratio
  Bus Selector1 : BusSelector  OutputSignals=accl
  Bus Selector2 : BusSelector  OutputSignals=limit_decel_ratio_cnt
  Constant : Constant  OutDataTypeStr=single
  Constant1 : Constant  OutDataTypeStr=single
  Divide : Product  Inputs=*/
  Product : Product
  Saturation : Saturate  UpperLimit=1  LowerLimit=0
  Switch : Switch  Criteria=u2 ~= 0  SaturateOnIntegerOverflow=off  InputSameDT=off
  ff_accl : Outport
  cnt_delay_accl_ratio : Outport  Port=2
  cnt_delay_decel_ratio : Outport  Port=3
  wires:
  Product/1 -> ff_accl/1
  Bus Selector2/1 -> Switch/1, Switch/2  "<limit_decel_ratio_cnt>"
  Add/1 -> cnt_delay_decel_ratio/1, Divide/1
  Divide/1 -> Saturation/1
  Saturation/1 -> Product/2
  ego/1 -> Bus Selector/1, Bus Selector1/1
  Constant/1 -> Add/2
  Bus Selector1/1 -> Product/1  "<accl>"
  tgt/1 -> Bus Selector2/1
  Bus Selector/1 -> Add/1  "<cnt_delay_decel_ratio>"
  Bus Selector/2 -> cnt_delay_accl_ratio/1  "<cnt_delay_accl_ratio>"
  Switch/1 -> Divide/2
  Constant1/1 -> Switch/3

== system mpc_tgt_calc/decel_ratio/If Action Subsystem2 ==
  ego : Inport
  Action Port : ActionPort  ActionPortLabel=else
  Bus Selector : BusSelector  OutputSignals=accl,cnt_delay_accl_ratio,cnt_delay_decel_ratio
  ff_accl : Outport
  cnt_delay_accl_ratio : Outport  Port=2
  cnt_delay_decel_ratio : Outport  Port=3
  wires:
  ego/1 -> Bus Selector/1
  Bus Selector/1 -> ff_accl/1  "<accl>"
  Bus Selector/2 -> cnt_delay_accl_ratio/1  "<cnt_delay_accl_ratio>"
  Bus Selector/3 -> cnt_delay_decel_ratio/1  "<cnt_delay_decel_ratio>"

== system mpc_tgt_calc/kanayama_ctrl_method1/Subsystem ==
  ego : Inport
  x_e : Inport  Port=2
  y_e : Inport  Port=3
  theta_e : Inport  Port=4
  tgt : Inport  Port=5
  Add : Sum
  Add1 : Sum
  Bus Selector : BusSelector  OutputSignals=v,w
  Bus Selector1 : BusSelector  OutputSignals=kanayama_gain.k_x,kanayama_gain.k_y,kanayama_gain.k_theta
  Cos : Trigonometry  Operator=cos
  Data Type Conversion : DataTypeConversion  OutDataTypeStr=single  SaturateOnIntegerOverflow=off  RndMeth=Floor
  Data Type Conversion1 : DataTypeConversion  OutDataTypeStr=single  SaturateOnIntegerOverflow=off  RndMeth=Floor
  Product : Product
  Product1 : Product
  Product2 : Product
  Scope : Scope
      settings: DataLoggingVariableName=ScopeData2
  v : Outport
  w : Outport  Port=2
  diff_y : Outport  Port=3
  wires:
  ego/1 -> Bus Selector/1
  tgt/1 -> Bus Selector1/1
  Bus Selector1/1 -> [k_x]  "<k_x>"
  Bus Selector1/2 -> [k_y]  "<k_y>"
  Bus Selector1/3 -> [k_theta]  "<k_theta>"
  Bus Selector/1 -> [ideal_v]  "<v>"
  Bus Selector/2 -> [ideal_w]  "<w>"
  [ideal_v] -> Product/1
  Cos/1 -> Product/2
  Product/1 -> Add/1
  Product1/1 -> Add/2
  [k_x] -> Product1/1
  [ideal_w] -> Add1/1
  Add/1 -> Data Type Conversion/1
  Data Type Conversion/1 -> v/1
  theta_e/1 -> Scope/1, Cos/1
  Add1/1 -> Data Type Conversion1/1
  Data Type Conversion1/1 -> w/1
  x_e/1 -> Product1/2
  Product2/1 -> Add1/2
  y_e/1 -> diff_y/1, Product2/2
  [k_y] -> Product2/1

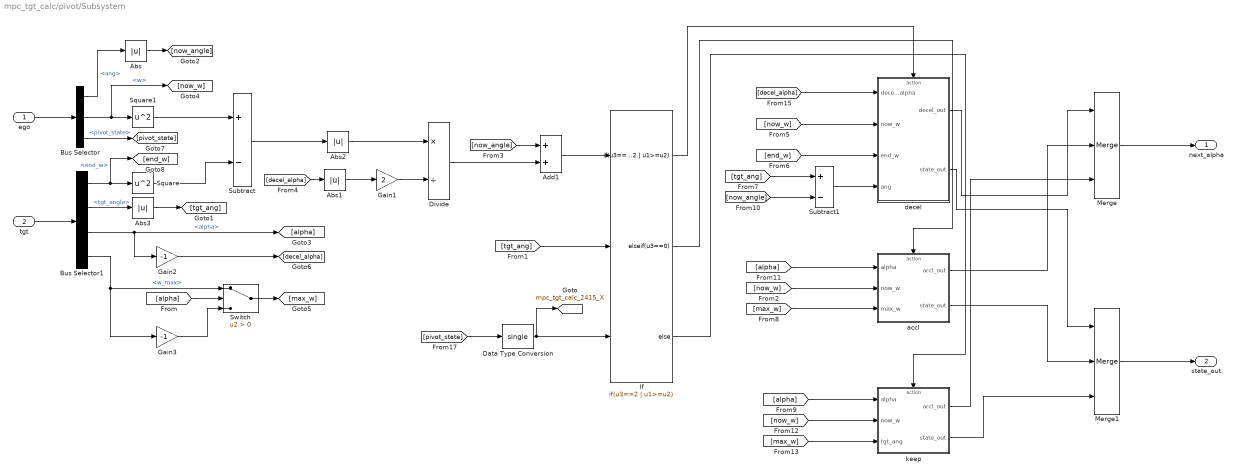
== system mpc_tgt_calc/pivot/Subsystem ==
  ego : Inport
  tgt : Inport  Port=2
  Abs{,1..3} (4 alike) : Abs  SaturateOnIntegerOverflow=off
  Add1 : Sum
  Bus Selector : BusSelector  OutputSignals=ang,w,pivot_state
  Bus Selector1 : BusSelector  OutputSignals=end_w,tgt_angle,alpha,w_max
  Data Type Conversion : DataTypeConversion  OutDataTypeStr=single  SaturateOnIntegerOverflow=off  RndMeth=Floor
  Divide : Product  Inputs=*/
  Gain1 : Gain  Gain=2
  Gain2 : Gain  Gain=-1
  Gain3 : Gain  Gain=-1
  If : If  NumInputs=3  IfExpression=u3==2 | u1>=u2  ElseIfExpressions=u3==0
  Merge : Merge  Inputs=3
  Merge1 : Merge  Inputs=3
  Square : Math  Operator=square
  Square1 : Math  Operator=square
  Subtract : Sum  Inputs=+-
  Subtract1 : Sum  Inputs=+-
  Switch : Switch  Criteria=u2 > Threshold  SaturateOnIntegerOverflow=off  InputSameDT=off
  accl : Subsystem  TreatAsAtomicUnit=on
  decel : Subsystem  TreatAsAtomicUnit=on
  keep : Subsystem  TreatAsAtomicUnit=on
  next_alpha : Outport
  state_out : Outport  Port=2
  tag scope: mpc_tgt_calc_2415_X=global
  wires:
  ego/1 -> Bus Selector/1
  Subtract/1 -> Abs2/1
  Divide/1 -> Add1/2
  [now_angle] -> Add1/1
  Abs1/1 -> Gain1/1
  Abs2/1 -> Divide/1
  [decel_alpha] -> Abs1/1
  Gain1/1 -> Divide/2
  tgt/1 -> Bus Selector1/1
  Bus Selector1/1 -> [end_w], Square/1  "<end_w>"
  Square/1 -> Subtract/2
  Square1/1 -> Subtract/1
  Bus Selector/3 -> [pivot_state]  "<pivot_state>"
  Bus Selector/2 -> [now_w], Square1/1  "<w>"
  Bus Selector/1 -> Abs/1  "<ang>"
  Bus Selector1/2 -> Abs3/1  "<tgt_angle>"
  Bus Selector1/3 -> Gain2/1, [alpha]  "<alpha>"
  Gain2/1 -> [decel_alpha]
  Switch/1 -> [max_w]
  [alpha] -> Switch/2
  Bus Selector1/4 -> Gain3/1, Switch/1  "<w_max>"
  Gain3/1 -> Switch/3
  [pivot_state] -> Data Type Conversion/1
  Data Type Conversion/1 -> If/3, [mpc_tgt_calc_2415_X]
  [tgt_ang] -> If/2
  Add1/1 -> If/1
  keep/2(state_out) -> Merge1/3
  decel/1(decel_out) -> Merge/1
  [max_w] -> keep/3(tgt_ang)
  accl/1(accl_out) -> Merge/2
  [now_w] -> keep/2(now_w)
  [decel_alpha] -> decel/1(decel_alpha)
  [now_w] -> decel/2(now_w)
  [now_angle] -> Subtract1/2
  [tgt_ang] -> Subtract1/1
  [now_w] -> accl/2(now_w)
  accl/2(state_out) -> Merge1/2
  If/2 -> accl/Action
  keep/1(accl_out) -> Merge/3
  [max_w] -> accl/3(max_w)
  [alpha] -> keep/1(alpha)
  If/3 -> keep/Action
  [end_w] -> decel/3(end_w)
  decel/2(state_out) -> Merge1/1
  Merge1/1 -> state_out/1
  Subtract1/1 -> decel/4(ang)
  If/1 -> decel/Action
  Merge/1 -> next_alpha/1
  [alpha] -> accl/1(alpha)
  Abs/1 -> [now_angle]
  Abs3/1 -> [tgt_ang]

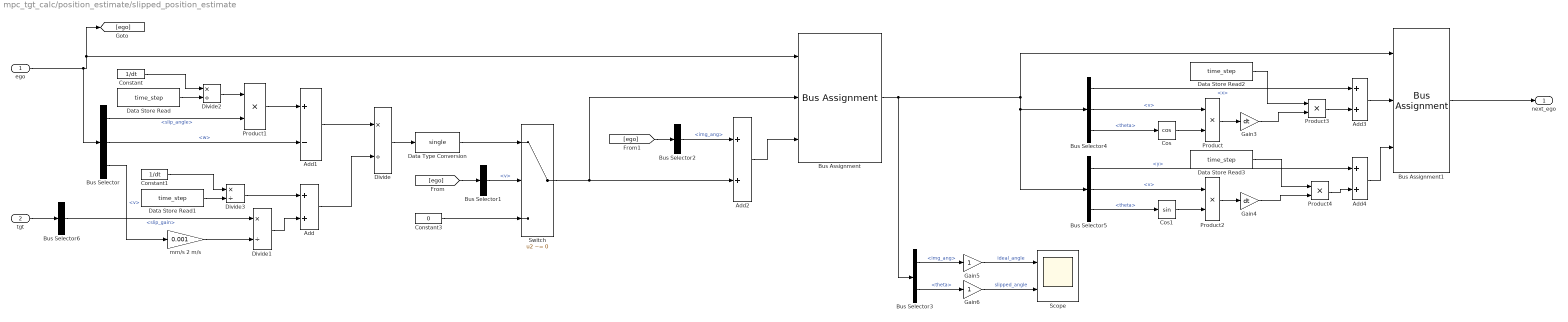
== system mpc_tgt_calc/position_estimate/slipped_position_estimate ==
  ego : Inport
  tgt : Inport  Port=2
  Add{,2..4} (4 alike) : Sum
  Add1 : Sum  Inputs=+-
  Bus Assignment : BusAssignment  AssignedSignals=slip_point.slip_angle,slip_point.theta
  Bus Assignment1 : BusAssignment  AssignedSignals=slip_point.x,slip_point.y
  Bus Selector : BusSelector  OutputSignals=slip_point.slip_angle,slip_point.w,v
  Bus Selector1 : BusSelector  OutputSignals=v
  Bus Selector2 : BusSelector  OutputSignals=img_ang
  Bus Selector3 : BusSelector  OutputSignals=img_ang,slip_point.theta
  Bus Selector4 : BusSelector  OutputSignals=slip_point.x,v,slip_point.theta
  Bus Selector5 : BusSelector  OutputSignals=slip_point.y,v,slip_point.theta
  Bus Selector6 : BusSelector  OutputSignals=slip_gain
  Constant : Constant  Value=1/dt  OutDataTypeStr=single
  Constant1 : Constant  Value=1/dt  OutDataTypeStr=single
  Constant3 : Constant  Value=0  OutDataTypeStr=single
  Cos : Trigonometry  Operator=cos
  Cos1 : Trigonometry
  Data Store Read{,1..3} (4 alike) : DataStoreRead  DataStoreName=time_step  IndexOptions=Index vector (dialog)  Indices=1  OutputSizes=1
  Data Type Conversion : DataTypeConversion  OutDataTypeStr=single  SaturateOnIntegerOverflow=off  RndMeth=Floor
  Divide{,1..3} (4 alike) : Product  Inputs=*/
  Gain3 : Gain  Gain=dt
  Gain4 : Gain  Gain=dt
  Gain5 : Gain
  Gain6 : Gain
  Product{,1..4} (5 alike) : Product
  Scope : Scope  NumInputPorts=2
      settings: ActiveDisplayYMinimum=-0.39272  ActiveDisplayYMaximum=3.5345
  Switch : Switch  Criteria=u2 ~= 0  SaturateOnIntegerOverflow=off  InputSameDT=off
  mm/s 2 m/s : Gain  Gain=0.001
  next_ego : Outport
  wires:
  ego/1 -> Bus Selector/1, Bus Assignment/1, [ego]
  Constant/1 -> Divide2/1
  Constant1/1 -> Divide3/1
  Divide3/1 -> Add/1
  Divide1/1 -> Add/2
  Add1/1 -> Divide/1
  Add/1 -> Divide/2
  Bus Selector/2 -> Add1/2  "<w>"
  Product1/1 -> Add1/1
  Divide2/1 -> Product1/1
  Bus Selector/1 -> Product1/2  "<slip_angle>"
  Bus Selector/3 -> mm/s 2 m/s/1  "<v>"
  Divide/1 -> Data Type Conversion/1
  mm/s 2 m/s/1 -> Divide1/2
  Data Type Conversion/1 -> Switch/1
  Switch/1 -> Bus Assignment/2, Add2/2
  Constant3/1 -> Switch/3
  [ego] -> Bus Selector1/1
  Bus Selector1/1 -> Switch/2  "<v>"
  Bus Selector2/1 -> Add2/1  "<img_ang>"
  [ego] -> Bus Selector2/1
  Add2/1 -> Bus Assignment/3
  Bus Selector3/1 -> Gain5/1  "<img_ang>"
  Bus Selector3/2 -> Gain6/1  "<theta>"
  Product2/1 -> Gain4/1
  Bus Selector5/1 -> Add4/1  "<y>"
  Bus Assignment/1 -> Bus Selector3/1, Bus Selector4/1, Bus Selector5/1, Bus Assignment1/1
  Bus Selector4/1 -> Add3/1  "<x>"
  Add3/1 -> Bus Assignment1/2
  Add4/1 -> Bus Assignment1/3
  Bus Selector5/3 -> Cos1/1  "<theta>"
  Bus Selector5/2 -> Product2/1  "<v>"
  Bus Selector4/2 -> Product/1  "<v>"
  Product/1 -> Gain3/1
  Cos/1 -> Product/2
  Bus Selector4/3 -> Cos/1  "<theta>"
  Cos1/1 -> Product2/2
  Bus Assignment1/1 -> next_ego/1
  Gain5/1 -> Scope/1  "ideal_angle"
  Gain6/1 -> Scope/2  "slipped_angle"
  tgt/1 -> Bus Selector6/1
  Bus Selector6/1 -> Divide1/1  "<slip_gain>"
  Data Store Read/1 -> Divide2/2
  Data Store Read1/1 -> Divide3/2
  Data Store Read2/1 -> Product3/1
  Product3/1 -> Add3/2
  Gain3/1 -> Product3/2
  Data Store Read3/1 -> Product4/1
  Product4/1 -> Add4/2
  Gain4/1 -> Product4/2
